simulink model "Simulacion_1"  (R2021b)
settings: Solver=VariableStepAuto  StartTime=0.0  StopTime=0.07  FixedStep=1000  MaxStep=0.0001  MinStep=0.00001  RelTol=1e-3
libraries: fl_lib x18, nesl_utility x10
settings Model: SnapshotBufferSize=1000  Creator=Roberto  LastModifiedBy=Roberto

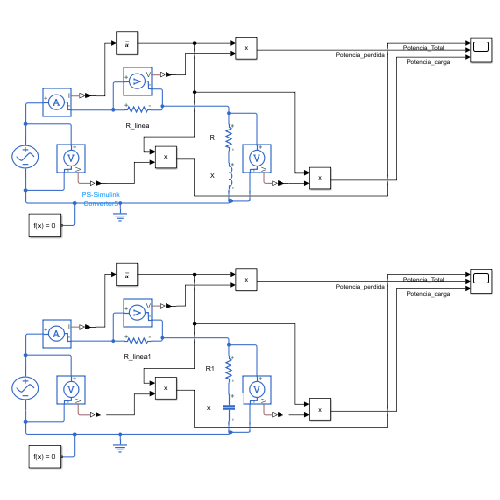
[thumbnail: Simulink's stored preview of the top-level diagram]
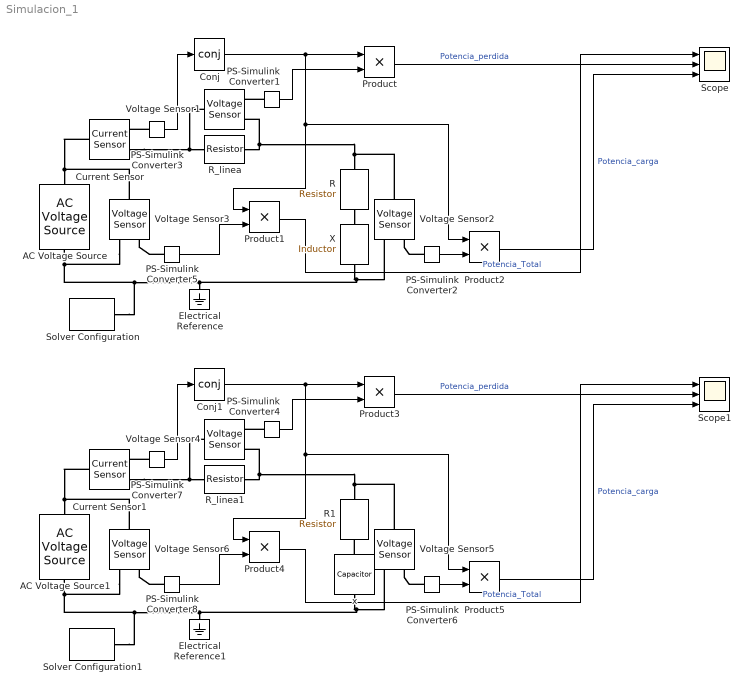
== system Simulacion_1 ==
  AC Voltage Source : fl_lib/Electrical/Electrical Sources/AC Voltage Source  amp=100 V  shift=0 deg  frequency=60 Hz  omega=0 rad/s
  AC Voltage Source1 : fl_lib/Electrical/Electrical Sources/AC Voltage Source  amp=100 V  shift=0 deg  frequency=60 Hz  omega=0 rad/s
  Conj : Math  Operator=conj  SaturateOnIntegerOverflow=on
  Conj1 : Math  Operator=conj  SaturateOnIntegerOverflow=on
  Current Sensor : fl_lib/Electrical/Electrical Sensors/Current Sensor
  Current Sensor1 : fl_lib/Electrical/Electrical Sensors/Current Sensor
  Electrical Reference : fl_lib/Electrical/Electrical Elements/Electrical Reference
  Electrical Reference1 : fl_lib/Electrical/Electrical Elements/Electrical Reference
  PS-Simulink Converter{1..8} (8 alike) : nesl_utility/PS-Simulink Converter  PhysicalDomain=network_engine_domain  SubClassName=ps_output  LeftPortType=input  RightPortType=output  PseudoPeriodic=off  Frequencies=[]  Unit=inherit  AffineConversion=off
      settings: SourceProductBaseCode=PW,SS
  Product{,1..5} (6 alike) : Product
  R : fl_lib/Electrical/Electrical Elements/Resistor  R=2 Ohm  i_specify=off  i_priority=None  i=0 A  i_nominal_specify=off  i_nominal_unit=A  i_nominal_value=1  v_specify=off  v_priority=None  v=0 V  v_nominal_specify=off  v_nominal_unit=V  v_nominal_value=1
  R1 : fl_lib/Electrical/Electrical Elements/Resistor  R=2 Ohm  i_specify=off  i_priority=None  i=0 A  i_nominal_specify=off  i_nominal_unit=A  i_nominal_value=1  v_specify=off  v_priority=None  v=0 V  v_nominal_specify=off  v_nominal_unit=V  v_nominal_value=1
  R_linea : fl_lib/Electrical/Electrical Elements/Resistor  R=0.5 Ohm  i_specify=off  i_priority=None  i=0 A  i_nominal_specify=off  i_nominal_unit=A  i_nominal_value=1  v_specify=off  v_priority=None  v=0 V  v_nominal_specify=off  v_nominal_unit=V  v_nominal_value=1
  R_linea1 : fl_lib/Electrical/Electrical Elements/Resistor  R=0.5 Ohm  i_specify=off  i_priority=None  i=0 A  i_nominal_specify=off  i_nominal_unit=A  i_nominal_value=1  v_specify=off  v_priority=None  v=0 V  v_nominal_specify=off  v_nominal_unit=V  v_nominal_value=1
  Scope : Scope  NumInputPorts=3
  Scope1 : Scope  NumInputPorts=3
  Solver Configuration : nesl_utility/Solver Configuration  PhysicalDomain=network_engine_domain  SubClassName=solver  LeftPortType=input  RightPortType=generic  Tones=[]  Harmonics=[]  SimulateNoise=off  Profile=off  UseLocalSampling=off  EnableSwitchedLinearOptims=on  FrequencyDomain=off  UseCCode=off  RelTol=0.001  AbsTol=1e-06  MinStep=1e-09  ToWorkspace=off  RevertToSquareIcSolve=off  NumHomotopyIterations=100  PhasorMode=off  PhasorModeNumHarmonics=1  DoDC=off  ResidualTolerance=1e-09  UseLocalSolver=off  LocalSolverChoice=NE_BACKWARD_EULER_ADVANCER  LocalSolverSampleTime=0.001  DoFixedCost=off  MaxNonlinIter=3  MaxModeIter=2  ComputeImpulses=off  ImpulseIterations=2  LinearAlgebra=auto  EquationFormulation=NE_TIME_EF  DelaysMemoryBudget=1024  AutomaticFiltering=on  FilteringTimeConstant=0.001  PartitionStorageMethod=AS_NEEDED  PartitionMemoryBudget=1024  PartitionMethod=ROBUST
      settings: SourceProductBaseCode=PW,SS
  Solver Configuration1 : nesl_utility/Solver Configuration  PhysicalDomain=network_engine_domain  SubClassName=solver  LeftPortType=input  RightPortType=generic  Tones=[]  Harmonics=[]  SimulateNoise=off  Profile=off  UseLocalSampling=off  EnableSwitchedLinearOptims=on  FrequencyDomain=off  UseCCode=off  RelTol=0.001  AbsTol=1e-06  MinStep=1e-09  ToWorkspace=off  RevertToSquareIcSolve=off  NumHomotopyIterations=100  PhasorMode=off  PhasorModeNumHarmonics=1  DoDC=off  ResidualTolerance=1e-09  UseLocalSolver=off  LocalSolverChoice=NE_BACKWARD_EULER_ADVANCER  LocalSolverSampleTime=0.001  DoFixedCost=off  MaxNonlinIter=3  MaxModeIter=2  ComputeImpulses=off  ImpulseIterations=2  LinearAlgebra=auto  EquationFormulation=NE_TIME_EF  DelaysMemoryBudget=1024  AutomaticFiltering=on  FilteringTimeConstant=0.001  PartitionStorageMethod=AS_NEEDED  PartitionMemoryBudget=1024  PartitionMethod=ROBUST
      settings: SourceProductBaseCode=PW,SS
  Voltage Sensor{1..6} (6 alike) : fl_lib/Electrical/Electrical Sensors/Voltage Sensor
  X : fl_lib/Electrical/Electrical Elements/Inductor  l=L H  r=0 Ohm  g=1e-9 1/Ohm  i_specify=off  i_priority=None  i=0 A  i_nominal_specify=off  i_nominal_unit=A  i_nominal_value=1  v_specify=off  v_priority=None  v=0 V  v_nominal_specify=off  v_nominal_unit=V  v_nominal_value=1  i_L_specify=off  i_L_priority=High  i_L=0 A  i_L_nominal_specify=off  i_L_nominal_unit=A  i_L_nominal_value=1
  x : fl_lib/Electrical/Electrical Elements/Capacitor  c=C F  r=1e-6 Ohm  g=0 1/Ohm  i_specify=off  i_priority=None  i=0 A  i_nominal_specify=off  i_nominal_unit=A  i_nominal_value=1  v_specify=off  v_priority=None  v=0 V  v_nominal_specify=off  v_nominal_unit=V  v_nominal_value=1  vc_specify=off  vc_priority=High  vc=0 V  vc_nominal_specify=off  vc_nominal_unit=V  vc_nominal_value=1
  wires:
  Conj/1 -> Product2/1, Product1/1, Product/1
  PS-Simulink Converter3/1 -> Conj/1
  PS-Simulink Converter2/1 -> Product2/2
  PS-Simulink Converter5/1 -> Product1/2
  Product2/1 -> Scope/3  "Potencia_carga"
  PS-Simulink Converter1/1 -> Product/2
  Product/1 -> Scope/2  "Potencia_perdida"
  Product1/1 -> Scope/1  "Potencia_Total"
  Product4/1 -> Scope1/1  "Potencia_Total"
  Conj1/1 -> Product5/1, Product4/1, Product3/1
  Product5/1 -> Scope1/3  "Potencia_carga"
  Product3/1 -> Scope1/2  "Potencia_perdida"
  PS-Simulink Converter4/1 -> Product3/2
  PS-Simulink Converter8/1 -> Product4/2
  PS-Simulink Converter6/1 -> Product5/2
  PS-Simulink Converter7/1 -> Conj1/1
  connections:
  R/RConn1 -- X/LConn1
  R_linea/RConn1 -- R/LConn1 -- Voltage Sensor2/LConn1 -- Voltage Sensor1/RConn2
  Current Sensor/LConn1 -- Voltage Sensor3/LConn1 -- AC Voltage Source/LConn1
  Current Sensor/RConn2 -- Voltage Sensor1/LConn1 -- R_linea/LConn1
  X/RConn1 -- Solver Configuration/RConn1 -- Voltage Sensor3/RConn2 -- AC Voltage Source/RConn1 -- Electrical Reference/LConn1 -- Voltage Sensor2/RConn2
  PS-Simulink Converter1/LConn1 -- Voltage Sensor1/RConn1
  PS-Simulink Converter2/LConn1 -- Voltage Sensor2/RConn1
  PS-Simulink Converter3/LConn1 -- Current Sensor/RConn1
  PS-Simulink Converter5/LConn1 -- Voltage Sensor3/RConn1
  Solver Configuration1/RConn1 -- x/RConn1 -- Voltage Sensor5/RConn2 -- Electrical Reference1/LConn1 -- Voltage Sensor6/RConn2 -- AC Voltage Source1/RConn1
  Current Sensor1/RConn2 -- Voltage Sensor4/LConn1 -- R_linea1/LConn1
  Current Sensor1/LConn1 -- Voltage Sensor6/LConn1 -- AC Voltage Source1/LConn1
  R_linea1/RConn1 -- R1/LConn1 -- Voltage Sensor5/LConn1 -- Voltage Sensor4/RConn2
  PS-Simulink Converter4/LConn1 -- Voltage Sensor4/RConn1
  PS-Simulink Converter6/LConn1 -- Voltage Sensor5/RConn1
  x/LConn1 -- R1/RConn1
  PS-Simulink Converter8/LConn1 -- Voltage Sensor6/RConn1
  PS-Simulink Converter7/LConn1 -- Current Sensor1/RConn1
